simulink model "Example5_Calibrating_The_AR_Drone_Model"  (R2016a)
settings: configuration reference "AR_Drone_ConfigSet" (kept outside this file)
libraries: AR_Drone_Sensors x1
settings Model: DataDictionary=ArDroneDataDictionary.sldd  SimulationMode=external  ExtModeTrigDuration=100000  Creator=sannem  LastModifiedBy=sannem
settings ConfigSetRef: DDName=ArDroneDataDictionary.sldd

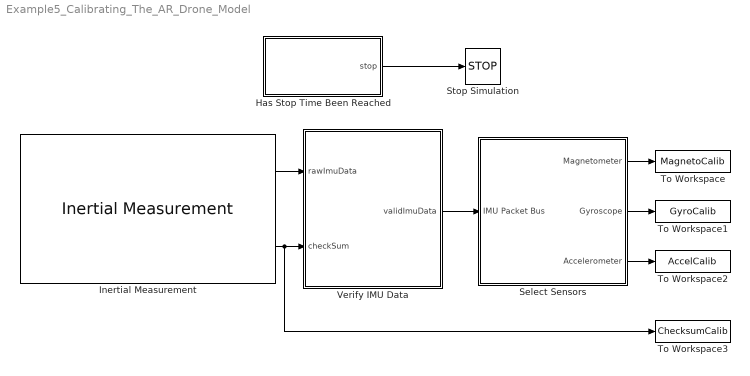
== system Example5_Calibrating_The_AR_Drone_Model ==
  Has Stop Time Been Reached : MATLAB Function  TreatAsAtomicUnit=on  SystemSampleTime=sampleTime  mask{stopTime=5, sampleTime=1/200}
      mask prompts: stopTime "Stop time [s]"; sampleTime "Sample time [s]"
      mask help: This block will keep track of the run time of a model. The default output is "0" with the output changing to "1" if the run time exceeds the user specified stop time.
  Inertial Measurement : AR_Drone_Sensors/Inertial Measurement  Ts=1/200
  Select Sensors : Subsystem
  Stop Simulation : Stop
  To Workspace : ToWorkspace  VariableName=MagnetoCalib  SaveFormat=Structure With Time  SampleTime=-1
  To Workspace1 : ToWorkspace  VariableName=GyroCalib  SaveFormat=Structure With Time  SampleTime=-1
  To Workspace2 : ToWorkspace  VariableName=AccelCalib  SaveFormat=Structure With Time  SampleTime=-1
  To Workspace3 : ToWorkspace  VariableName=ChecksumCalib  SaveFormat=Structure With Time  SampleTime=-1
  Verify IMU Data : MATLAB Function  TreatAsAtomicUnit=on
  wires:
  Has Stop Time Been Reached/1(stop) -> Stop Simulation/1
  Verify IMU Data/1(validImuData) -> Select Sensors/1(IMU Packet Bus)
  Select Sensors/1(Magnetometer) -> To Workspace/1
  Select Sensors/2(Gyroscope) -> To Workspace1/1
  Select Sensors/3(Accelerometer) -> To Workspace2/1
  Inertial Measurement/2 -> Verify IMU Data/2(checkSum), To Workspace3/1
  Inertial Measurement/1 -> Verify IMU Data/1(rawImuData)

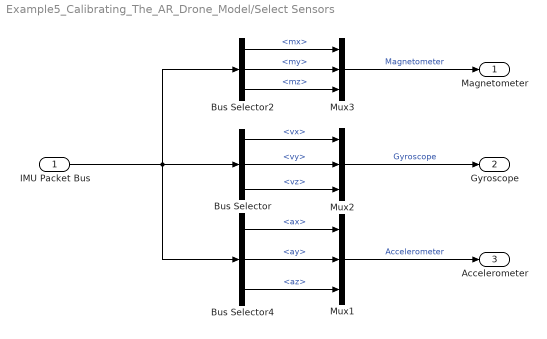
== system Example5_Calibrating_The_AR_Drone_Model/Select Sensors ==
  IMU Packet Bus : Inport  OutDataTypeStr=Bus: IMU_Packets
  Bus Selector : BusSelector  OutputSignals=vx,vy,vz
  Bus Selector2 : BusSelector  OutputSignals=mx,my,mz
  Bus Selector4 : BusSelector  OutputSignals=ax,ay,az
  Mux1 : Mux  Inputs=3
  Mux2 : Mux  Inputs=3
  Mux3 : Mux  Inputs=3
  Magnetometer : Outport
  Gyroscope : Outport  Port=2
  Accelerometer : Outport  Port=3
  wires:
  Bus Selector/3 -> Mux2/3  "<vz>"
  Bus Selector/2 -> Mux2/2  "<vy>"
  Bus Selector/1 -> Mux2/1  "<vx>"
  Bus Selector2/3 -> Mux3/3  "<mz>"
  Bus Selector2/2 -> Mux3/2  "<my>"
  Bus Selector2/1 -> Mux3/1  "<mx>"
  Bus Selector4/3 -> Mux1/3  "<az>"
  Bus Selector4/2 -> Mux1/2  "<ay>"
  Bus Selector4/1 -> Mux1/1  "<ax>"
  IMU Packet Bus/1 -> Bus Selector4/1, Bus Selector/1, Bus Selector2/1
  Mux1/1 -> Accelerometer/1  "Accelerometer"
  Mux2/1 -> Gyroscope/1  "Gyroscope"
  Mux3/1 -> Magnetometer/1  "Magnetometer"

== matlab function Example5_Calibrating_The_AR_Drone_Model/Verify IMU Data ==
  data: rawImuData input Bus: IMU_Packets; validImuData output Bus: IMU_Packets; checkSum input
function validImuData = verifyImuData(rawImuData, checkSum)
%#codegen

%% When the checksum fails the corresponding packet will contain bad data.
% If the checksum passes again it can still be that the packet will be the
% same as the previously received bad packet, this function checks whether
% the checksum fails and keeps outputting the last good packet untill a new
% packet arrives which is different from the packet which failed.

% %% v1 using full packet comparison

% persistent storedGoodPacket
% if isempty(storedGoodPacket)
%     storedGoodPacket = rawImuData;
% end
% 
% persistent storedBadPacket
% if isempty(storedBadPacket)
%     storedBadPacket = rawImuData;
% end
% 
% if checkSum == 0 % checksum failed, save the bad packet to compare with future packets
%     validImuData = storedGoodPacket;
%     storedBadPacket = rawImuData;
% else             % checksum passed but could still be bad data
%     if isequal(rawImuData,storedBadPacket) % the new data is still the bad data
%         validImuData = storedGoodPacket;
%     else         % the new packet is not equal to the bad packet, update good packet to new packet
%         storedGoodPacket = rawImuData; 
%         validImuData = rawImuData;
%     end
% end

%% v2 using only checksum comparison

persistent storedGoodPacket
if isempty(storedGoodPacket)
    storedGoodPacket = rawImuData;
end

persistent storedBadChecksum
if isempty(storedBadChecksum)
    storedBadChecksum = rawImuData.chksum;
end

if checkSum == 0 % checksum flag failed, save the bad packet checksum to compare with future packets
    validImuData = storedGoodPacket;
    storedBadChecksum = rawImuData.chksum;
else             % checksum flag passed but could still be bad data
    if isequal(rawImuData.chksum,storedBadChecksum) % the new data is still the bad data
        validImuData = storedGoodPacket;
    else         % the new packet is not equal to the bad packet, update good packet to new packet
        storedGoodPacket = rawImuData; 
        validImuData = rawImuData;
    end
end

== matlab function Example5_Calibrating_The_AR_Drone_Model/Has Stop Time Been Reached ==
  data: stop output; stopTime parameter; sampleTime parameter
function stop = stopTimeReached(stopTime,sampleTime)
%#codegen

% persistent variable which keeps track of the total run time
persistent runTime
if isempty(runTime)
    runTime = sampleTime
else
    runTime = runTime + sampleTime;
end

stop = 0;
% verify whether the stop time is reached
if runTime > stopTime
    stop = 1;
end
